simulink model "untitled2"  (R2019b)
settings: Solver=VariableStepAuto  StartTime=0.0  StopTime=10.0  RelTol=1e-3
undefined symbols (not defined in the file or in its folder): sigbuilder_block
libraries: simulink x1
settings Model: Creator=YJR  LastModifiedBy=YJR

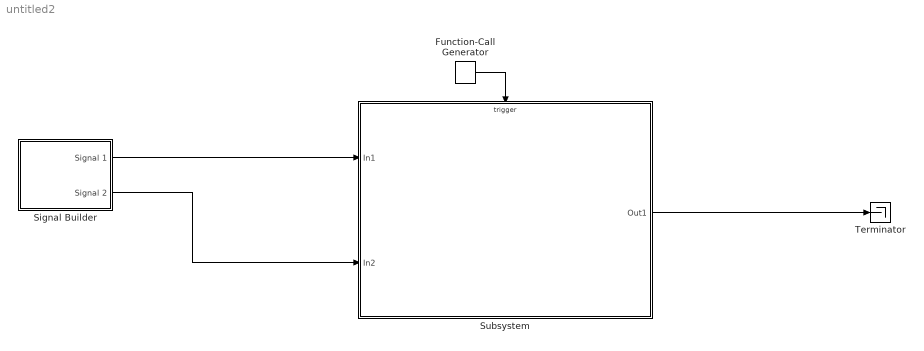
== system untitled2 ==
  Function-Call Generator : simulink/Ports & Subsystems/Function-Call Generator  sample_time=0.01  numberOfIterations=1
  Signal Builder : Subsystem  Tag=STV Subsys  LoadFcn=sigbuilder_block('load');  StartFcn=sigbuilder_block('start');  StopFcn=sigbuilder_block('stop');  ClipboardFcn=sigbuilder_block('clipboard');  mask(Sigbuilder block){tuvar=[0:10]}
      mask help: Simulink:masks:SigbuilderBlock_MD
      mask init:
      | if ~strcmp(get_param(bdroot(gcbh),'SimulationStatus'),'stopped') tuvar = sigbuilder_block('maskInit'); end
      settings: CopyFcn=sigbuilder_block('copy');  DeleteFcn=sigbuilder_block('delete');  ModelCloseFcn=sigbuilder_block('modelClose');  PreSaveFcn=sigbuilder_block('preSave');  PauseFcn=sigbuilder_block('pause');  ContinueFcn=sigbuilder_block('continue');  NameChangeFcn=sigbuilder_block('namechange');  OpenFcn=sigbuilder_block('open',[437.6 199.2 550.4 400 ]);  CloseFcn=sigbuilder_block('close');
      mask Display: plot(0, 0, 100, 100,[2, 2, 32, 32, 2], [68, 8, 8, 68, 68],[32, 2], [38, 38], [32, 19, 2],[53, 60, 44], [32, 17, 17, 2],[16, 16, 31, 31]);txt = getActiveGroup(gcbh);text(2, 100, txt,'verticalAlignment', 'top');
  Subsystem : Subsystem
  Terminator : Terminator
  wires:
  Signal Builder/1(Signal 1) -> Subsystem/1(In1)
  Signal Builder/2(Signal 2) -> Subsystem/2(In2)
  Subsystem/1(Out1) -> Terminator/1
  Function-Call Generator/1 -> Subsystem/Trigger

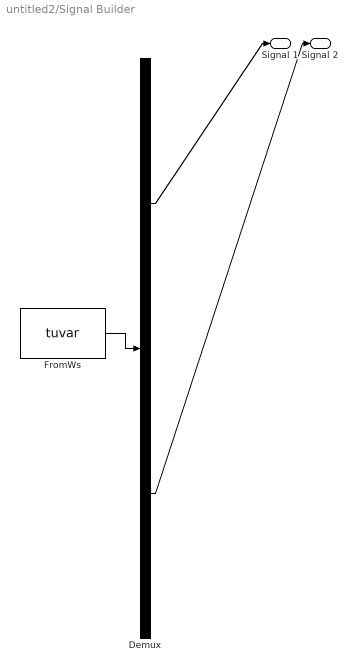
== system untitled2/Signal Builder ==
  Demux : Demux  Tag=STV Demux  Outputs=2
  FromWs : FromWorkspace  Tag=STV FromWs  VariableName=tuvar  SampleTime=0
      SigBuilderData=|
      | common.afterFinalStr = 'Extrapolate'
      | common.sampleTime = 0
      | dataSet.timeRange = [0 10]
      | dataSet.name = 'Group 1'
      | sbobj.Groups.Name = 'Group 1'
      | sbobj.Groups.Signals(1).Name = 'Signal 1'
      | sbobj.Groups.Signals(1).XData = [0 1.25 2.5 2.5 3.75 3.75 5 6.25 7.5 7.5 8.75 8.75 10]
      | sbobj.Groups.Signals(1).YData = [0 0 0 1 1 0 0 0 0 1 1 0 0]
      | sbobj.Groups.Signals(2).Name = 'Signal 2'
      | sbobj.Groups.Signals(2).XData = [0 1.25 2.5 2.5 3.75 3.75 5 5 6.25 6.25 7.5 8.75 10]
      | sbobj.Groups.Signals(2).YData = [0 0 0 1 1 0 0 1 1 0 0 0 0]
  Signal 1 : Outport  Tag=STV Outport
  Signal 2 : Outport  Tag=STV Outport  Port=2
  wires:
  FromWs/1 -> Demux/1
  Demux/1 -> Signal 1/1
  Demux/2 -> Signal 2/1

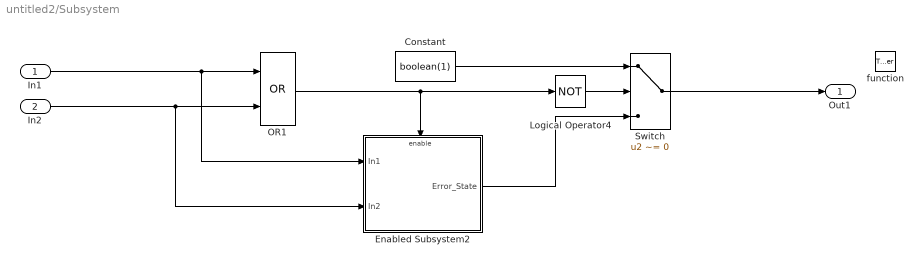
== system untitled2/Subsystem ==
  In1 : Inport
  In2 : Inport  Port=2
  function : TriggerPort  TriggerType=function-call  VariantControl=Variant
  Constant : Constant  Value=boolean(1)
  Enabled Subsystem2 : Subsystem  TreatAsAtomicUnit=on
  Logical Operator4 : Logic  Operator=NOT  AllPortsSameDT=off  OutDataTypeStr=boolean
  OR1 : Logic  Operator=OR  AllPortsSameDT=off  OutDataTypeStr=boolean
  Switch : Switch  Criteria=u2 ~= 0
  Out1 : Outport
  wires:
  In1/1 -> Enabled Subsystem2/1(In1), OR1/1
  OR1/1 -> Logical Operator4/1, Enabled Subsystem2/Enable
  In2/1 -> Enabled Subsystem2/2(In2), OR1/2
  Logical Operator4/1 -> Switch/2
  Constant/1 -> Switch/1
  Enabled Subsystem2/1(Error_State) -> Switch/3
  Switch/1 -> Out1/1

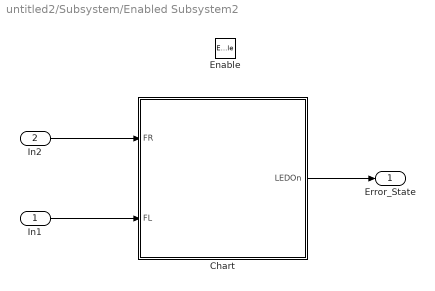
== system untitled2/Subsystem/Enabled Subsystem2 ==
  In1 : Inport
  In2 : Inport  Port=2
  Enable : EnablePort
  Chart : Stateflow chart  BlockKeywords=__PRM__SERIALIZED__DATA__:Stateflow Chart,Stateflow Diagram  TreatAsAtomicUnit=on
  Error_State : Outport
  wires:
  In1/1 -> Chart/2(FL)
  In2/1 -> Chart/1(FR)
  Chart/1(LEDOn) -> Error_State/1

== stateflow chart untitled2/Subsystem/Enabled Subsystem2/Chart ==
  state Init
  state StateA
    state LEDON
      en:
      LEDOn=0;
    state LEDOFF
      en:
      LEDOn=1;
    StateA.LEDON -> StateA.LEDOFF : after(0.8,sec)
    (default) -> StateA.LEDON
    StateA.LEDOFF -> StateA.LEDON : after(0.8,sec)
  state StateB
    state LEDON
      en:
      LEDOn=0;
    state LEDOFF
      en:
      LEDOn=1;
    StateB.LEDON -> StateB.LEDOFF : after(0.4,sec)
    (default) -> StateB.LEDON
    StateB.LEDOFF -> StateB.LEDON : after(0.4,sec)
  state StateC
    state LEDON
      en:
      LEDOn=0;
    state LEDOFF
      en:
      LEDOn=1;
    StateC.LEDON -> StateC.LEDOFF : after(0.1,sec)
    (default) -> StateC.LEDON
    StateC.LEDOFF -> StateC.LEDON : after(0.1,sec)
  (default) -> Init
  Init -> StateA [order 1] : [FL&&~FR]
  StateA -> Init : [~FL||FR]
  Init -> StateB [order 2] : [~FL&&FR]
  StateB -> Init : [FL||~FR]
  Init -> StateC [order 3] : [FL&&FR]
  StateC -> Init : [~FL||~FR]
  data: LEDOn output; FR input; FL input
